simulink model "Estimator_Simulink_trial2"  (R2019a)
settings: Solver=ode4  StartTime=0.0  StopTime=9000  FixedStep=.01  RelTol=1e-3
values from neighbouring files (symbols this model uses):
  A1 = A(1,1)    [BatteryModel_1stOrder_Youla.m]    (also in Estimator_Simulink_driver.m)
  A2 = A(2,2)    [BatteryModel_1stOrder_Youla.m]    (also in Estimator_Simulink_driver.m)
  B1 = B(1,1)    [BatteryModel_1stOrder_Youla.m]    (also in Estimator_Simulink_driver.m)
  B2 = B(2,1)    [BatteryModel_1stOrder_Youla.m]    (also in Estimator_Simulink_driver.m)
  D = -R0    (= -0.1)    [BatteryModel_1stOrder_Youla.m]    (also in Estimator_Simulink_driver.m = [-R0]; battery_equivalent_circuit_model_KF.m = -0.01)
undefined symbols (not defined in the file or in its folder): den, num
libraries: dspsrcs4 x3, simulink x1, dspstat3 x1
settings Model: Creator=felip  LastModifiedBy=Indiana

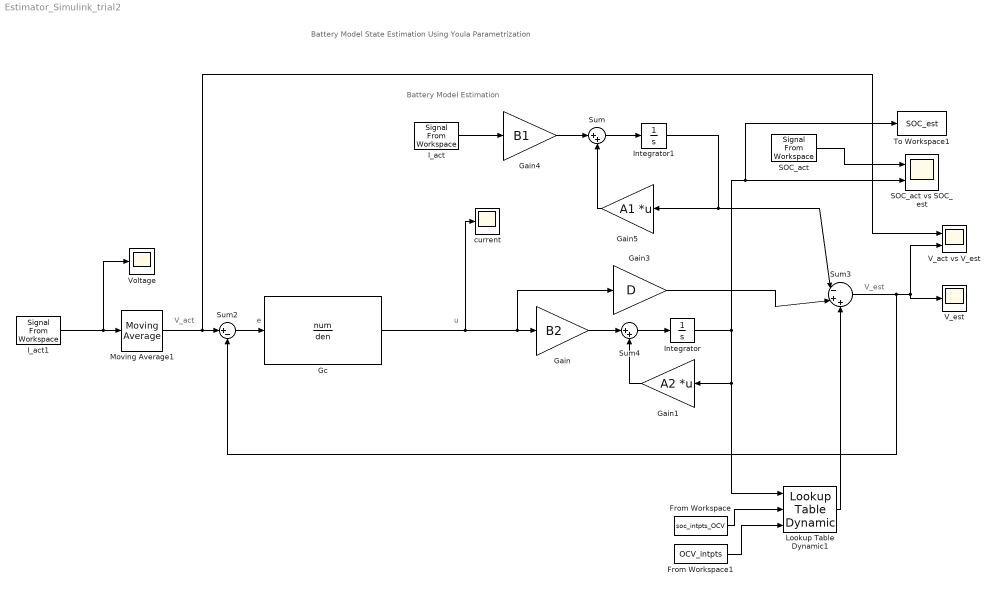
== system Estimator_Simulink_trial2 ==
  note: V_act
  note: u
  note: e
  note: V_est
  note: Battery Model Estimation
  note: Battery Model State Estimation Using Youla Parametrization
  From Workspace : FromWorkspace  VariableName=soc_intpts_OCV  SampleTime=0
  From Workspace1 : FromWorkspace  VariableName=OCV_intpts  SampleTime=0
  Gain : Gain  Gain=B2
  Gain1 : Gain  Gain=A2  Multiplication=Matrix(K*u)
  Gain3 : Gain  Gain=D
  Gain4 : Gain  Gain=B1
  Gain5 : Gain  Gain=A1  Multiplication=Matrix(K*u)
  Gc : TransferFcn  Numerator=num  Denominator=den
  I_act : dspsrcs4/Signal From Workspace  X=I  Ts=.1  nsamps=1  OutputAfterFinalValue=Setting to zero  ignoreOrWarnInputAndFrameLengths=off  OutputFrames=off
  I_act1 : dspsrcs4/Signal From Workspace  X=V  Ts=.1  nsamps=1  OutputAfterFinalValue=Setting to zero  ignoreOrWarnInputAndFrameLengths=off  OutputFrames=off
  Integrator : Integrator  InitialCondition=1
  Integrator1 : Integrator
  Lookup Table Dynamic1 : simulink/Lookup Tables/Lookup Table Dynamic  LookUpMeth=Interpolation-Use End Values  OutDataType=fixdt('double')  OutScaling=[]  OutputDataTypeScalingMode=Specify via dialog  OutDataTypeStr=double  DoSatur=off
      settings: SourceProductName=Simulink
  Moving Average1 : dspstat3/Moving Average  Method=Sliding window  ForgettingFactorPort=off  SpecifyWindowLength=on  WindowLength=25  ForgettingFactor=0.9  SimulateUsing=Code generation
  SOC_act : dspsrcs4/Signal From Workspace  X=SOC_act  Ts=.1  nsamps=1  OutputAfterFinalValue=Setting to zero  ignoreOrWarnInputAndFrameLengths=off  OutputFrames=off
  SOC_act vs SOC_est : Scope  NumInputPorts=2
  Sum : Sum  Inputs=|++
  Sum2 : Sum  Inputs=|+-
  Sum3 : Sum  Inputs=|-++
  Sum4 : Sum  Inputs=|++
  To Workspace1 : ToWorkspace  VariableName=SOC_est  SampleTime=-1
      settings: Save2DSignal=2-D array (concatenate along first dimension)
  V_act vs V_est : Scope  NumInputPorts=2
  "V_est " : Scope
  Voltage : Scope
  "current " : Scope
  wires:
  Sum4/1 -> Integrator/1
  Gain1/1 -> Sum4/2
  Moving Average1/1 -> V_act vs V_est/1, Sum2/1
  Gain/1 -> Sum4/1
  Gc/1 -> Gain3/1, Gain/1, "current "/1
  SOC_act/1 -> SOC_act vs SOC_est/1
  Sum2/1 -> Gc/1
  Sum3/1 -> "V_est "/1, V_act vs V_est/2, Sum2/2
  I_act/1 -> Gain4/1
  Gain4/1 -> Sum/1
  Gain5/1 -> Sum/2
  Sum/1 -> Integrator1/1
  Gain3/1 -> Sum3/2
  Integrator1/1 -> Gain5/1, Sum3/1
  Integrator/1 -> Lookup Table Dynamic1/1, Gain1/1, To Workspace1/1, SOC_act vs SOC_est/2
  I_act1/1 -> Voltage/1, Moving Average1/1
  From Workspace1/1 -> Lookup Table Dynamic1/3
  From Workspace/1 -> Lookup Table Dynamic1/2
  Lookup Table Dynamic1/1 -> Sum3/3
